simulink model "minor_pjct"  (Simulink 7.2)
settings: Solver=ode45  StartTime=0.0  StopTime=1  RelTol=1e-3
undefined symbols (not defined in the file): D1, Delta
libraries: powerlib x29, powerlib_extras x3
settings Model: Creator=Electrical 2  LastModifiedBy=user
settings OptimizationCC: InitFltsAndDblsToZero=on

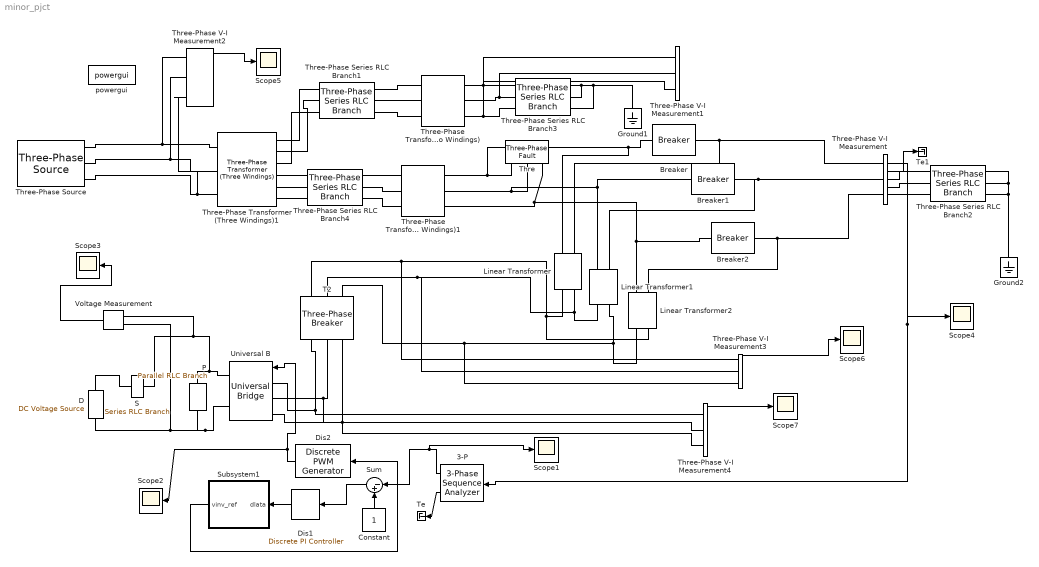
== system minor_pjct ==
  3-P : powerlib_extras/Measurements/3-Phase Sequence Analyzer  Orientation=left  DialogController=POWERSYS.PowerSysDialog  SystemSampleTime=-1  f1=50  n=1  seq=Positive
  Breaker : powerlib/Elements/Breaker  DialogController=POWERSYS.PowerSysDialog  SystemSampleTime=-1  BreakerResistance=0.01  InitialState=1  SnubberResistance=1e6  SnubberCapacitance=inf  SwitchingTimes=[0.4 0.6]  External=off  Measurements=None  MoreParameters=off  NoBreakLoop=off
  Breaker1 : powerlib/Elements/Breaker  DialogController=POWERSYS.PowerSysDialog  SystemSampleTime=-1  BreakerResistance=0.01  InitialState=1  SnubberResistance=1e6  SnubberCapacitance=inf  SwitchingTimes=[0.4 0.6]  External=off  Measurements=None  MoreParameters=off  NoBreakLoop=off
  Breaker2 : powerlib/Elements/Breaker  DialogController=POWERSYS.PowerSysDialog  SystemSampleTime=-1  BreakerResistance=0.01  InitialState=1  SnubberResistance=1e6  SnubberCapacitance=inf  SwitchingTimes=[0.4 0.6]  External=off  Measurements=None  MoreParameters=off  NoBreakLoop=off
  Constant : Constant  Orientation=up  OutDataType=sfix(16)  OutScaling=2^0
  D : powerlib/Electrical Sources/DC Voltage Source  Orientation=up  DialogController=POWERSYS.PowerSysDialog  SystemSampleTime=-1  Amplitude=4e3  Measurements=None
  Dis1 : powerlib_extras/Discrete  Control Blocks/Discrete PI Controller  Orientation=left  DialogController=POWERSYS.PowerSysDialog  SystemSampleTime=-1  Kp=0.5  Ki=50  Par_Limits=[1e6 -1e6]  Init=0  Ts=50e-6
  Dis2 : powerlib_extras/Discrete  Control Blocks/Discrete PWM Generator  Orientation=left  DialogController=POWERSYS.PowerSysDialog  SystemSampleTime=-1  GeneratorMode="3-arm  bridge (6 pulses)"  Fc=1080  Ts=5e-6  Internal=off  mIndex=0.4  Freq=60  Phase=0
  Ground1 : powerlib/Elements/Ground  Orientation=down  DialogController=POWERSYS.PowerSysDialog  PhysicalDomain=powersysdomain  SubClassName=unknown  LeftPortType=p1  RightPortType=p1  LConnTagsString=a
  Ground2 : powerlib/Elements/Ground  Orientation=down  DialogController=POWERSYS.PowerSysDialog  PhysicalDomain=powersysdomain  SubClassName=unknown  LeftPortType=p1  RightPortType=p1  LConnTagsString=a
  Linear Transformer : powerlib/Elements/Linear Transformer  Orientation=down  DialogController=POWERSYS.PowerSysDialog  PhysicalDomain=powersysdomain  SubClassName=unknown  LeftPortType=p1  RightPortType=p1  LConnTagsString=a|b  RConnTagsString=A|B  UNITS=pu  NominalPower=[ 250e6 50 ]  winding1="[11e3  0.002  0.08 ]"  winding2="[9e3  0.002  0.08 ]"  ThreeWindings=off  winding3=[ 60e3 0.005 0.02 ]  RmLm=[ 500 500 ]  Measurements=None  DataType=off
  Linear Transformer1 : powerlib/Elements/Linear Transformer  Orientation=down  DialogController=POWERSYS.PowerSysDialog  PhysicalDomain=powersysdomain  SubClassName=unknown  LeftPortType=p1  RightPortType=p1  LConnTagsString=a|b  RConnTagsString=A|B  UNITS=pu  NominalPower=[ 250e6 50 ]  winding1="[11e3  0.002  0.08 ]"  winding2="[9e3  0.002  0.08 ]"  ThreeWindings=off  winding3=[ 60e3 0.005 0.02 ]  RmLm=[ 500 500 ]  Measurements=None  DataType=off
  Linear Transformer2 : powerlib/Elements/Linear Transformer  Orientation=down  DialogController=POWERSYS.PowerSysDialog  PhysicalDomain=powersysdomain  SubClassName=unknown  LeftPortType=p1  RightPortType=p1  LConnTagsString=a|b  RConnTagsString=A|B  UNITS=pu  NominalPower=[ 250e6 50 ]  winding1="[11e3  0.002  0.08 ]"  winding2="[9e3  0.002  0.08 ]"  ThreeWindings=off  winding3=[ 60e3 0.005 0.02 ]  RmLm=[ 500 500 ]  Measurements=None  DataType=off
  P : powerlib/Elements/Parallel RLC Branch  Orientation=down  DialogController=POWERSYS.PowerSysDialog  PhysicalDomain=powersysdomain  SubClassName=unknown  LeftPortType=p1  RightPortType=p1  LConnTagsString=a  RConnTagsString=__new0  BranchType=C  Resistance=[]  Inductance=[]  SetiL0=off  InitialCurrent=0  Capacitance=750e-6  Setx0=off  InitialVoltage=0  Measurements=Branch voltage and current
  S : powerlib/Elements/Series RLC Branch  DialogController=POWERSYS.PowerSysDialog  PhysicalDomain=powersysdomain  SubClassName=unknown  LeftPortType=p1  RightPortType=p1  LConnTagsString=__new0  RConnTagsString=__new0  BranchType=R  Resistance=10  Inductance=1e-3  SetiL0=off  InitialCurrent=0  Capacitance=1e-6  Setx0=off  InitialVoltage=0  Measurements=None
  Scope{1..7} (7 alike) : Scope
      Scope1 settings: YMin=0.15  YMax=1
      Scope2 settings: YMin=0.78  YMax=1
      Scope3 settings: YMin=-50  YMax=750  SaveName=ScopeData3
      Scope4 settings: YMin=-0.3  YMax=0.3  SaveName=ScopeData5
      Scope5 settings: YMin=-1.2  YMax=1.2  SaveName=ScopeData4
      Scope6 settings: TimeRange=0.005138304153271767  YMin=-0.07  YMax=0.07  SaveName=ScopeData6
      Scope7 settings: YMin=-0.6  YMax=0.6  SaveName=ScopeData7
  Subsystem1 : Subsystem  Orientation=left
  Sum : Sum  Orientation=left  Inputs=|-+  OutDataType=sfix(16)  OutScaling=2^0
  T2 : powerlib/Elements/Three-Phase Breaker  Orientation=down  DialogController=POWERSYS.PowerSysDialog  SystemSampleTime=-1  InitialState=closed  SwitchA=off  SwitchB=off  SwitchC=off  SwitchTimes=[0.4 0.6]  External=off  BreakerResistance=0.001  SnubberResistance=1e6  SnubberCapacitance=inf  Measurements=None
  Te : Terminator
  Te1 : Terminator
  Thre : powerlib/Elements/Three-Phase Fault  Orientation=up  DialogController=POWERSYS.PowerSysDialog  SystemSampleTime=-1  FaultA=on  FaultB=on  FaultC=on  FaultResistance=0.66  GroundFault=on  GroundResistance=0.4  External=off  SwitchStatus=[1 0]  SwitchTimes=[ 0.4 0.6]  InitialStates=[0 0 1]  SnubberResistance=1e6  SnubberCapacitance=inf  Measurements=None
  Three-Phase Series RLC Branch1 : powerlib/Elements/Three-Phase Series RLC Branch  DialogController=POWERSYS.PowerSysDialog  PhysicalDomain=powersysdomain  SubClassName=unknown  LeftPortType=p1  RightPortType=p1  LConnTagsString=A|B|C  RConnTagsString=A|B|C  BranchType=RL  Resistance=.05  Inductance=0.4806  Capacitance=1e-6  Measurements=None
  Three-Phase Series RLC Branch2 : powerlib/Elements/Three-Phase Series RLC Branch  DialogController=POWERSYS.PowerSysDialog  PhysicalDomain=powersysdomain  SubClassName=unknown  LeftPortType=p1  RightPortType=p1  LConnTagsString=A|B|C  RConnTagsString=A|B|C  BranchType=RL  Resistance=0.1  Inductance=.1926  Capacitance=1e-6  Measurements=Branch voltages
  Three-Phase Series RLC Branch3 : powerlib/Elements/Three-Phase Series RLC Branch  DialogController=POWERSYS.PowerSysDialog  PhysicalDomain=powersysdomain  SubClassName=unknown  LeftPortType=p1  RightPortType=p1  LConnTagsString=A|B|C  RConnTagsString=A|B|C  BranchType=R  Resistance=20  Inductance=1e-3  Capacitance=1e-6  Measurements=None
  Three-Phase Series RLC Branch4 : powerlib/Elements/Three-Phase Series RLC Branch  DialogController=POWERSYS.PowerSysDialog  PhysicalDomain=powersysdomain  SubClassName=unknown  LeftPortType=p1  RightPortType=p1  LConnTagsString=A|B|C  RConnTagsString=A|B|C  BranchType=RL  Resistance=0.001  Inductance=0.005  Capacitance=1e-6  Measurements=None
  Three-Phase Transformer (Three Windings)1 : powerlib/Elements/Three-Phase Transformer (Three Windings)  DialogController=POWERSYS.PowerSysDialog  SystemSampleTime=-1  Winding1Connection=Yg  UNITS=pu  NominalPower=[ 100e6 , 50 ]  Winding1=[13e3 , 0.002 , 0.08 ]  Winding2Connection=Delta (D1)  Winding2=[115e3 , 0.002 , 0.08 ]  Winding3Connection=Delta (D1)  Winding3=[115e3 , 0.002 , 0.08 ]  SetSaturation=off  Rm=500  Lm=500  Saturation=[ 0,0 ; 0.0024,1.2 ; 1.0,1.52 ]  Hysteresis=off  DataFile='hysteresis'  SetInitialFlux=off  InitialFluxes=[0.8 -0.8 0.7]  Measurements=None  MoreParameters=off  BreakLoop=off  DataType=off  TransfoNumber=0
  Three-Phase Transformer (Two Windings) : powerlib/Elements/Three-Phase Transformer (Two Windings)  DialogController=POWERSYS.PowerSysDialog  SystemSampleTime=-1  Winding1Connection=Delta (D1)  UNITS=pu  NominalPower=[ 250e6 , 50 ]  Winding1=[ 115e3 , 0.002 , 0.08 ]  Winding2Connection=Yg  Winding2=[ 11e3 , 0.002 , 0.08 ]  SetSaturation=off  Rm=500  Lm=500  Saturation=[ 0,0 ; 0.0024,1.2 ; 1.0,1.52 ]  Hysteresis=off  DataFile='hysteresis'  SetInitialFlux=off  InitialFluxes=[ 0.8 , -0.8 , 0.7 ]  Measurements=None  MoreParameters=off  BreakLoop=off  DataType=off  TransfoNumber=0
  Three-Phase Transformer (Two Windings)1 : powerlib/Elements/Three-Phase Transformer (Two Windings)  DialogController=POWERSYS.PowerSysDialog  SystemSampleTime=-1  Winding1Connection=Y  UNITS=pu  NominalPower=[ 250e6 , 50 ]  Winding1=[ 115e3 , 0.002 , 0.08 ]  Winding2Connection=Delta (D1)  Winding2=[ 11e3 , 0.002 , 0.08 ]  SetSaturation=off  Rm=500  Lm=500  Saturation=[ 0,0 ; 0.0024,1.2 ; 1.0,1.52 ]  Hysteresis=off  DataFile='hysteresis'  SetInitialFlux=off  InitialFluxes=[ 0.8 , -0.8 , 0.7 ]  Measurements=None  MoreParameters=off  BreakLoop=off  DataType=off  TransfoNumber=0
  Three-Phase V-I Measurement : powerlib/Measurements/Three-Phase V-I Measurement  DialogController=POWERSYS.PowerSysDialog  SystemSampleTime=-1  VoltageMeasurement=phase-to-ground  SetLabelV=off  LabelV=Vabc  Vpu=on  CurrentMeasurement=yes  SetLabelI=off  LabelI=Iabc  Ipu=on  Pbase=100e6  Vbase=11e3  OutputType=Complex  PhasorSimulation=off  PSBequivalent=0
  Three-Phase V-I Measurement1 : powerlib/Measurements/Three-Phase V-I Measurement  DialogController=POWERSYS.PowerSysDialog  SystemSampleTime=-1  VoltageMeasurement=phase-to-ground  SetLabelV=off  LabelV=Vabc  Vpu=on  CurrentMeasurement=yes  SetLabelI=off  LabelI=Iabc  Ipu=on  Pbase=100e6  Vbase=11e3  OutputType=Complex  PhasorSimulation=off  PSBequivalent=0
  Three-Phase V-I Measurement2 : powerlib/Measurements/Three-Phase V-I Measurement  DialogController=POWERSYS.PowerSysDialog  SystemSampleTime=-1  VoltageMeasurement=phase-to-ground  SetLabelV=off  LabelV=Vabc  Vpu=on  CurrentMeasurement=yes  SetLabelI=off  LabelI=Iabc  Ipu=on  Pbase=100e6  Vbase=11e3  OutputType=Complex  PhasorSimulation=off  PSBequivalent=0
  Three-Phase V-I Measurement3 : powerlib/Measurements/Three-Phase V-I Measurement  DialogController=POWERSYS.PowerSysDialog  SystemSampleTime=-1  VoltageMeasurement=phase-to-phase  SetLabelV=off  LabelV=Vabc  Vpu=on  CurrentMeasurement=yes  SetLabelI=off  LabelI=Iabc  Ipu=on  Pbase=100e6  Vbase=11e3  OutputType=Complex  PhasorSimulation=off  PSBequivalent=0
  Three-Phase V-I Measurement4 : powerlib/Measurements/Three-Phase V-I Measurement  DialogController=POWERSYS.PowerSysDialog  SystemSampleTime=-1  VoltageMeasurement=phase-to-phase  SetLabelV=off  LabelV=Vabc  Vpu=on  CurrentMeasurement=yes  SetLabelI=off  LabelI=Iabc  Ipu=on  Pbase=100e6  Vbase=11e3  OutputType=Complex  PhasorSimulation=off  PSBequivalent=0
  Three-Phase Source : powerlib/Electrical Sources/Three-Phase Source  DialogController=POWERSYS.PowerSysDialog  SystemSampleTime=-1  Voltage=13e3  PhaseAngle=0  Frequency=50  InternalConnection=Yg  SpecifyImpedance=off  Resistance=0.1  Inductance=0  ShortCircuitLevel=100e6  BaseVoltage=25e3  XRratio=7
  Universal B : powerlib/Power Electronics/Universal Bridge  Orientation=left  DialogController=POWERSYS.PowerSysDialog  SystemSampleTime=-1  Arms=3  SnubberResistance=1e5  SnubberCapacitance=inf  Device=IGBT / Diodes  Ron=1e-3  Lon=0  ForwardVoltages="[  0  0  ]"  ForwardVoltage=0  GTOparameters=[ 10e-6 , 20e-6 ]  IGBTparameters=[ 1e-6 , 2e-6 ]  Measurements=None  Measurements_2=None  converterType=Rectifier
      link override Uswitch: GotoTag=tp182559
  Voltage Measurement : powerlib/Measurements/Voltage Measurement  Orientation=left  DialogController=POWERSYS.PowerSysDialog  SystemSampleTime=-1  PhasorSimulation=off  OutputType=Complex  PSBequivalent=0
  powergui : powerlib/powergui  SystemSampleTime=-1  SimulationMode=Discrete  SampleTime=1e-5  frequency=60  SPID=off  DisableSnubberDevices=off  DisableRonSwitches=off  DisableVfSwitches=off  SwTol=0  Interpol=off  frequencyindice=50  echomessages=off  HookPort=off  FunctionMessages=off  EnableUseOfTLC=off  x0status=blocks  RestoreLinks=warning  Frange=[0:2:500]  Ylog=off  Xlog=on  ShowGrid=off  save=off  variable=ZData  ZoomFFT=on  StartTime=0.0  cycles=1  DisplayStyle=1  fundamental=60  FreqAxis=off  MaxFrequency=1000  frequencyindicesteady=1  RmsSteady=1  display=off  Ts=0  methode=off
  wires:
  Dis2/1 -> Universal B/1, Scope2/1
  3-P/2 -> Te/1
  3-P/1 -> Scope1/1, Sum/1
  Constant/1 -> Sum/2
  Sum/1 -> Dis1/1
  Dis1/1 -> Subsystem1/1(dlata)
  Subsystem1/1(vinv_ref) -> Dis2/1
  Voltage Measurement/1 -> Scope3/1
  Three-Phase V-I Measurement2/1 -> Scope5/1
  Three-Phase V-I Measurement/2 -> Te1/1
  Three-Phase V-I Measurement/1 -> 3-P/1, Scope4/1
  Three-Phase V-I Measurement4/1 -> Scope7/1
  Three-Phase V-I Measurement3/1 -> Scope6/1
  connections:
  Universal B/RConn1 -- Voltage Measurement/LConn1 -- S/RConn1 -- P/LConn1
  Voltage Measurement/LConn2 -- Universal B/RConn2 -- P/RConn1 -- D/LConn1
  Three-Phase Series RLC Branch3/RConn2 -- Three-Phase Series RLC Branch3/RConn1 -- Ground1/LConn1 -- Three-Phase Series RLC Branch3/RConn3
  Three-Phase V-I Measurement2/LConn1 -- Three-Phase Source/RConn1 -- Three-Phase Transformer (Three Windings)1/LConn1
  Three-Phase V-I Measurement2/LConn3 -- Three-Phase Source/RConn3 -- Three-Phase Transformer (Three Windings)1/LConn3
  Three-Phase V-I Measurement2/LConn2 -- Three-Phase Source/RConn2 -- Three-Phase Transformer (Three Windings)1/LConn2
  Three-Phase Series RLC Branch2/RConn2 -- Ground2/LConn1 -- Three-Phase Series RLC Branch2/RConn3 -- Three-Phase Series RLC Branch2/RConn1
  Linear Transformer2/RConn2 -- Linear Transformer/RConn1 -- T2/LConn1 -- Three-Phase V-I Measurement3/LConn1
  Linear Transformer1/RConn1 -- Linear Transformer/RConn2 -- T2/LConn2 -- Three-Phase V-I Measurement3/LConn2
  T2/LConn3 -- Linear Transformer2/RConn1 -- Linear Transformer1/RConn2 -- Three-Phase V-I Measurement3/LConn3
  Three-Phase Series RLC Branch4/RConn3 -- Three-Phase Transformer (Two Windings)1/LConn3
  Three-Phase Series RLC Branch4/LConn3 -- Three-Phase Transformer (Three Windings)1/RConn6
  Three-Phase Transformer (Three Windings)1/RConn5 -- Three-Phase Series RLC Branch4/LConn2
  Three-Phase Transformer (Two Windings)1/LConn2 -- Three-Phase Series RLC Branch4/RConn2
  Three-Phase Series RLC Branch2/LConn1 -- Three-Phase V-I Measurement/RConn1
  Three-Phase Transformer (Three Windings)1/RConn2 -- Three-Phase Series RLC Branch1/LConn2
  Three-Phase Series RLC Branch1/LConn3 -- Three-Phase Transformer (Three Windings)1/RConn3
  Three-Phase Series RLC Branch4/LConn1 -- Three-Phase Transformer (Three Windings)1/RConn4
  Three-Phase Transformer (Three Windings)1/RConn1 -- Three-Phase Series RLC Branch1/LConn1
  Three-Phase Series RLC Branch4/RConn1 -- Three-Phase Transformer (Two Windings)1/LConn1
  Three-Phase Transformer (Two Windings)/RConn3 -- Three-Phase Series RLC Branch3/LConn3 -- Three-Phase V-I Measurement1/LConn3
  Three-Phase Series RLC Branch3/LConn2 -- Three-Phase Transformer (Two Windings)/RConn2 -- Three-Phase V-I Measurement1/LConn2
  Three-Phase Transformer (Two Windings)/RConn1 -- Three-Phase Series RLC Branch3/LConn1 -- Three-Phase V-I Measurement1/LConn1
  Three-Phase Series RLC Branch1/RConn3 -- Three-Phase Transformer (Two Windings)/LConn3
  Three-Phase Series RLC Branch1/RConn2 -- Three-Phase Transformer (Two Windings)/LConn2
  Three-Phase Transformer (Two Windings)/LConn1 -- Three-Phase Series RLC Branch1/RConn1
  Three-Phase Series RLC Branch2/LConn3 -- Three-Phase V-I Measurement/RConn3
  Universal B/LConn2 -- T2/RConn2 -- Three-Phase V-I Measurement4/LConn2
  Universal B/LConn1 -- T2/RConn1 -- Three-Phase V-I Measurement4/LConn1
  Universal B/LConn3 -- T2/RConn3 -- Three-Phase V-I Measurement4/LConn3
  S/LConn1 -- D/RConn1
  Three-Phase V-I Measurement/RConn2 -- Three-Phase Series RLC Branch2/LConn2
  Linear Transformer2/LConn1 -- Breaker2/LConn1 -- Three-Phase Transformer (Two Windings)1/RConn3 -- Thre/LConn3
  Three-Phase V-I Measurement/LConn1 -- Breaker/RConn1 -- Linear Transformer/LConn2
  Three-Phase V-I Measurement/LConn2 -- Breaker1/RConn1 -- Linear Transformer1/LConn2
  Three-Phase V-I Measurement/LConn3 -- Breaker2/RConn1 -- Linear Transformer2/LConn2
  Three-Phase Transformer (Two Windings)1/RConn1 -- Thre/LConn1 -- Linear Transformer/LConn1 -- Breaker/LConn1
  Breaker1/LConn1 -- Linear Transformer1/LConn1 -- Three-Phase Transformer (Two Windings)1/RConn2 -- Thre/LConn2

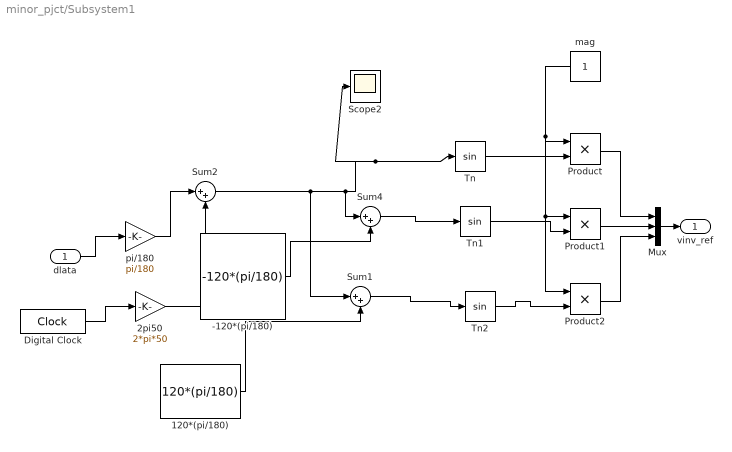
== system minor_pjct/Subsystem1 ==
  dlata : Inport  OutDataType=sfix(16)  OutScaling=2^0
  -120*(pi/180) : Constant  Value=-120*(pi/180)  OutDataType=sfix(16)  OutScaling=2^0
  120*(pi/180) : Constant  Value=120*(pi/180)  OutDataType=sfix(16)  OutScaling=2^0
  2pi50 : Gain  Gain=2*pi*50  ParameterDataType=sfix(16)  ParameterScaling=2^0  OutDataType=sfix(16)  OutScaling=2^0
  Digital Clock : DigitalClock  SampleTime=5e-6
  Mux : Mux  Inputs=3
  Product : Product  OutDataType=sfix(16)  OutScaling=2^0  RndMeth=Zero
  Product1 : Product  OutDataType=sfix(16)  OutScaling=2^0  RndMeth=Zero
  Product2 : Product  OutDataType=sfix(16)  OutScaling=2^0  RndMeth=Zero
  Scope2 : Scope
      settings: YMin=0  YMax=25  SaveName=ScopeData2
  Sum1 : Sum  Inputs=|++  OutDataType=sfix(16)  OutScaling=2^0
  Sum2 : Sum  Inputs=|++  OutDataType=sfix(16)  OutScaling=2^0
  Sum4 : Sum  Inputs=|++  OutDataType=sfix(16)  OutScaling=2^0
  Tn : Trigonometry
  Tn1 : Trigonometry
  Tn2 : Trigonometry
  mag : Constant  Orientation=left  OutDataType=sfix(16)  OutScaling=2^0
  pi/180 : Gain  Gain=pi/180  ParameterDataType=sfix(16)  ParameterScaling=2^0  OutDataType=sfix(16)  OutScaling=2^0
  vinv_ref : Outport  OutDataType=sfix(16)  OutScaling=2^0
  wires:
  mag/1 -> Product2/1, Product1/1, Product/1
  Tn2/1 -> Product2/2
  Sum2/1 -> Sum4/1, Tn/1, Scope2/1, Sum1/1
  Sum4/1 -> Tn1/1
  -120*(pi/180)/1 -> Sum4/2
  Sum1/1 -> Tn2/1
  120*(pi/180)/1 -> Sum1/2
  pi/180/1 -> Sum2/1
  2pi50/1 -> Sum2/2
  Digital Clock/1 -> 2pi50/1
  dlata/1 -> pi/180/1
  Product/1 -> Mux/1
  Product1/1 -> Mux/2
  Product2/1 -> Mux/3
  Mux/1 -> vinv_ref/1
  Tn/1 -> Product/2
  Tn1/1 -> Product1/2
